simulink model "test1"  (R2015a)
settings: Solver=ode3  StartTime=0.0  StopTime=inf  RelTol=1e-3
values from neighbouring files (symbols this model uses):
  simout = [12 12 12 12 13 12 12 12 12 11 11 11 ... (97 elements, 97x1)]    [test_data_set2.mat]    (also in test_dataset_3.mat = [11 11 11 11 11 11 11 11 10 10 10 10 ... (67 elements, 67x1))
libraries: legoev3lib x2
settings Model: SimulationMode=external  ExtModeTrigDuration=2  Creator=USER  LastModifiedBy=Keshav
settings OptimizationCC: OptimizeModelRefInitCode=on  LifeSpan=1
settings DebuggingCC: UnderspecifiedInitializationDetection=Classic  MergeDetectMultiDrivingBlocksExec=none
settings HardwareCC: ProdLargestAtomicInteger=Long  ProdLargestAtomicFloat=Float  ProdEndianess=LittleEndian  ProdHWDeviceType=ARM Compatible->ARM 9
settings RTWCC: SystemTargetFile=realtime.tlc  GenerateMakefile=off  TemplateMakefile=realtime.tmf  Description=Run on Target Hardware  RTWVerbose=off
settings ERTTargetCC: CombineOutputUpdateFcns=off  ERTSrcFileBannerTemplate=realtime_code_template.cgt  ERTHdrFileBannerTemplate=realtime_code_template.cgt  ERTDataSrcFileTemplate=realtime_code_template.cgt  ERTDataHdrFileTemplate=realtime_code_template.cgt  ERTCustomFileTemplate=realtime_file_process.tlc

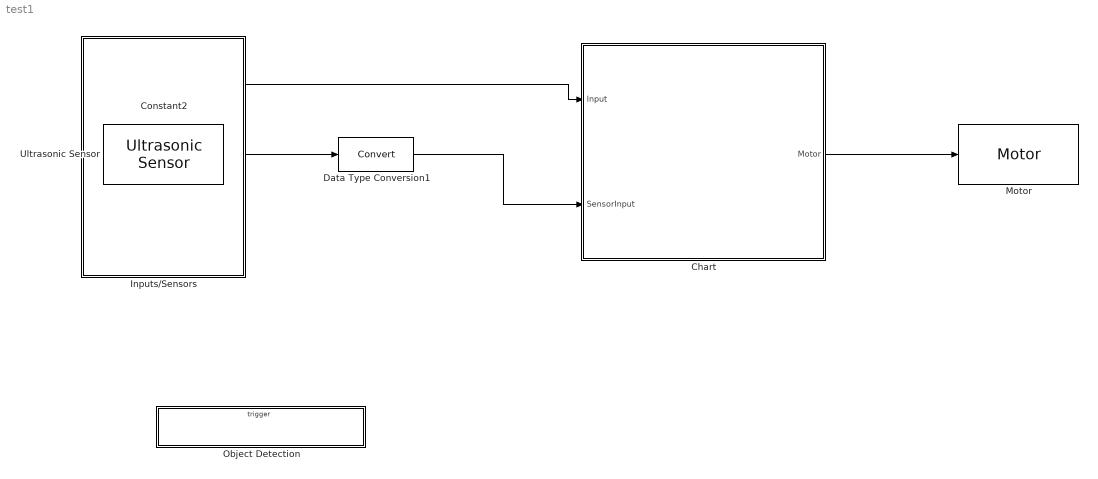
== system test1 ==
  Chart : Stateflow chart  TreatAsAtomicUnit=on
  Constant2 : Constant  Value=20
  Data Type Conversion1 : DataTypeConversion
  Inputs/Sensors : Subsystem
  Motor : legoev3lib/Motor  sportNumber=A  sstopAction=Brake
  Object Detection : Subsystem  TreatAsAtomicUnit=on
  Ultrasonic Sensor : legoev3lib/Ultrasonic Sensor  PortNumber=1  sampleTime=0.01
  wires:
  Ultrasonic Sensor/1 -> Data Type Conversion1/1
  Data Type Conversion1/1 -> Chart/2(SensorInput)
  Constant2/1 -> Chart/1(Input)
  Chart/1(Motor) -> Motor/1

== system test1/Inputs//Sensors ==

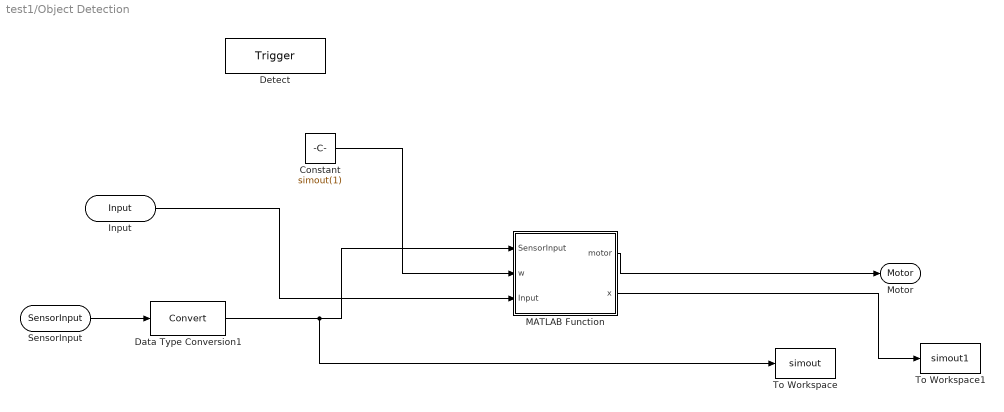
== system test1/Object Detection ==
  Detect : TriggerPort  TriggerType=function-call  IsSimulinkFunction=on  FunctionName=Detect
  Constant : Constant  Value=simout(1)
  Data Type Conversion1 : DataTypeConversion
  MATLAB Function : MATLAB Function  TreatAsAtomicUnit=on
  To Workspace : ToWorkspace  VariableName=simout  SampleTime=-1
  To Workspace1 : ToWorkspace  VariableName=simout1  SaveFormat=Timeseries  SampleTime=-1
  SensorInput : ArgIn  DisableCoverage=on  ArgumentName=SensorInput
  Input : ArgIn  DisableCoverage=on  Port=2  ArgumentName=Input
  Motor : ArgOut  DisableCoverage=on  ArgumentName=Motor
  wires:
  MATLAB Function/1(motor) -> Motor/1
  Constant/1 -> MATLAB Function/2(w)
  Input/1 -> MATLAB Function/3(Input)
  SensorInput/1 -> Data Type Conversion1/1
  Data Type Conversion1/1 -> To Workspace/1, MATLAB Function/1(SensorInput)
  MATLAB Function/2(x) -> To Workspace1/1

== matlab function test1/Object Detection/MATLAB Function ==
  data: SensorInput input; motor output; w input; Input input; x output
function [motor,x] = fcn(SensorInput,w,Input)
x=w;
if((SensorInput-x)>2)|| ((SensorInput-x)<-2)
    motor = 0;
elseif(SensorInput>4)&&(SensorInput<=20)
    motor = Input;
end
end

== stateflow chart test1/Chart ==
  (default) -> (junction 19) : {Motor = Detect(Input,SensorInput)}
  (junction 19) -> (junction 29)
  data: Input input; Motor output; SensorInput input
